simulink model "multirate"  (Simulink 7.0)
settings: Solver=ode3  SolverMode=SingleTasking  StartTime=0.0  StopTime=3  FixedStep=0.25  MaxStep=3  RelTol=1e-3
settings Model: Creator=dyblenko  LastModifiedBy=dyblenko

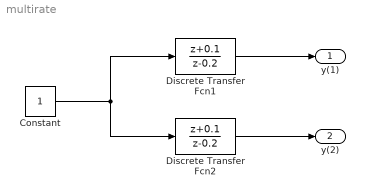
== system multirate ==
  Constant : Constant  OutDataType=sfix(16)  OutScaling=2^0
  Discrete Transfer Fcn1 : DiscreteTransferFcn  Numerator=[1 0.1]  Denominator=[1 -0.2]  SampleTime=0.75
  Discrete Transfer Fcn2 : DiscreteTransferFcn  Numerator=[1 0.1]  Denominator=[1 -0.2]  SampleTime=0.5
  y(1) : Outport  OutDataType=sfix(16)  OutScaling=2^0
  y(2) : Outport  Port=2  OutDataType=sfix(16)  OutScaling=2^0
  wires:
  Constant/1 -> Discrete Transfer Fcn1/1, Discrete Transfer Fcn2/1
  Discrete Transfer Fcn1/1 -> y(1)/1
  Discrete Transfer Fcn2/1 -> y(2)/1
